simulink model "vibration_harvester"  (R2025b)
settings: Solver=ode23tb  StartTime=0.0  StopTime=10  RelTol=1e-3  AbsTol=1e-6
values from neighbouring files (symbols this model uses):
  alpha = 0.15    [RegenVariables.mat]
  B = 0.05    [RegenVariables.mat]
  C1 = 2000    [RegenVariables.mat]
  C_boost = 0.00047    [RegenVariables.mat]
  C_buck = 0.00022    [RegenVariables.mat]
  cs = 1500    [RegenVariables.mat]
  D = 0.5    [RegenVariables.mat]
  ESR_boost = 3    [RegenVariables.mat]
  ESR_buck = 0.5    [RegenVariables.mat]
  eta = 0.98    [RegenVariables.mat]
  eta_bs = 0.9    [RegenVariables.mat]
  J = 0.01    [RegenVariables.mat]
  Ke = 0.5    [RegenVariables.mat]
  ks = 18000    [RegenVariables.mat]
  Kt = 0.5    [RegenVariables.mat]
  kt = 200000    [RegenVariables.mat]
  L_boost = 0.002    [RegenVariables.mat]
  L_buck = 0.001    [RegenVariables.mat]
  La = 0.005    [RegenVariables.mat]
  ms = 320    [RegenVariables.mat]
  mu = 45    [RegenVariables.mat]
  OCV0 = 3    [RegenVariables.mat]
  OCV_slope = 1.2    [RegenVariables.mat]
  p = 0.005    [RegenVariables.mat]
  Q_nom = 360000    [RegenVariables.mat]
  R0 = 0.05    [RegenVariables.mat]
  R1 = 0.02    [RegenVariables.mat]
  R_load = 50    [RegenVariables.mat]
  Ra = 2    [RegenVariables.mat]
  sigma = 0.002    [RegenVariables.mat]
  SOC0 = 0.5    [RegenVariables.mat]
  v = 20    [RegenVariables.mat]
  v_bat_init = 3.6    [RegenVariables.mat]
libraries: simulink x1
settings Model: NumberOfSteps=1000  Creator=khalid  LastModifiedBy=khalid
settings SolverCC: AutoScaleAbsTol=off

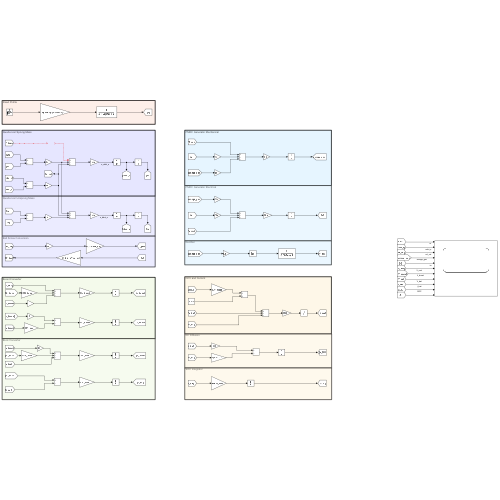
[thumbnail: Simulink's stored preview of the top-level diagram]
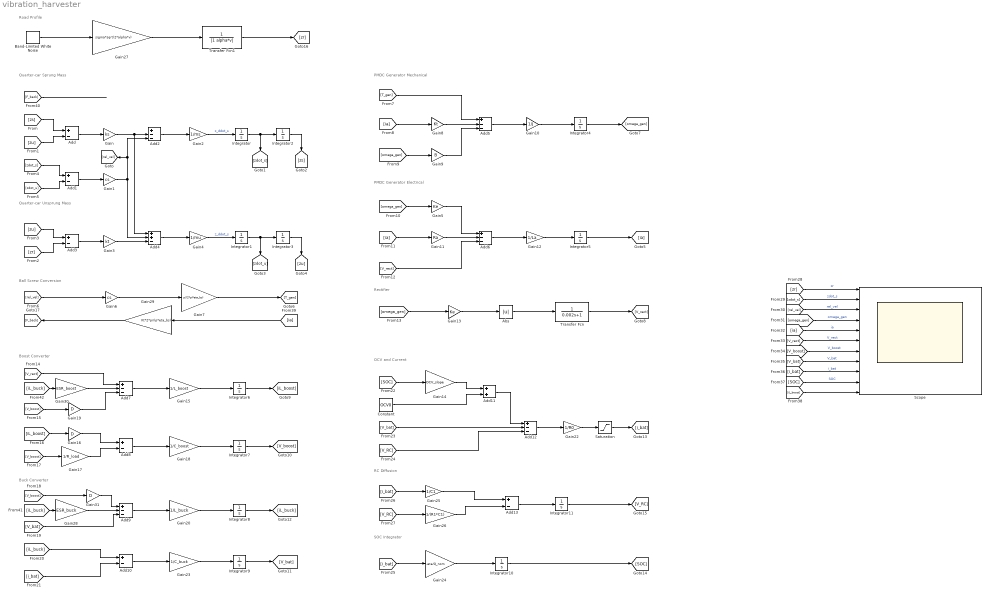
== system vibration_harvester ==
  note: Road Profile
  note: SOC Integrator
  note: RC Diffusion
  note: OCV and Current
  note: Boost Converter
  note: PMDC Generator Mechanical
  note: Ball Screw Conversion
  note: Quarter-car Unsprung Mass
  note: Quarter-car Sprung Mass
  note: PMDC Generator Electrical
  note: Rectifier
  note: Buck Converter
  Abs : Abs  SaturateOnIntegerOverflow=off
  Add{,1,3,8,10,13} (6 alike) : Sum  Inputs=+-
  Add11 : Sum
  Add{2,5..7,9,12} (6 alike) : Sum  Inputs=+--
  Add4 : Sum  Inputs=++-
  Band-Limited White Noise : simulink/Sources/Band-Limited White Noise  Cov=[1]  Ts=0.001  seed=[23341]
  Constant : Constant  Value=OCV0
  Gain : Gain  Gain=ks
  Gain1 : Gain  Gain=cs
  Gain10 : Gain  Gain=1/J
  Gain11 : Gain  Gain=Ra
  Gain12 : Gain  Gain=1/La
  Gain13 : Gain  Gain=Ke
  Gain14 : Gain  Gain=OCV_slope
  Gain15 : Gain  Gain=1/L_boost
  Gain16 : Gain  Gain=D
  Gain17 : Gain  Gain=1/R_load
  Gain18 : Gain  Gain=1/C_boost
  Gain19 : Gain  Gain=D
  Gain2 : Gain  Gain=1/ms
  Gain20 : Gain  Gain=1/L_buck
  Gain22 : Gain  Gain=1/R0
  Gain23 : Gain  Gain=1/C_buck
  Gain24 : Gain  Gain=-eta/Q_nom
  Gain25 : Gain  Gain=1/C1
  Gain26 : Gain  Gain=1/(R1*C1)
  Gain27 : Gain  Gain=sigma*sqrt(2*alpha*v)
  Gain28 : Gain  Gain=ESR_buck
  Gain29 : Gain  Gain=Kt*2*pi/(p*eta_bs)
  Gain3 : Gain  Gain=kt
  Gain30 : Gain  Gain=ESR_boost
  Gain31 : Gain  Gain=D
  Gain4 : Gain  Gain=1/mu
  Gain5 : Gain  Gain=Ke
  Gain6 : Gain  Gain=cs
  Gain7 : Gain  Gain=p/(2*pi*eta_bs)
  Gain8 : Gain  Gain=Kt
  Gain9 : Gain  Gain=B
  Integrator{,1..7,11} (9 alike) : Integrator
  Integrator10 : Integrator  InitialCondition=SOC0  UpperSaturationLimit=1  LowerSaturationLimit=0
  Integrator8 : Integrator  LowerSaturationLimit=0
  Integrator9 : Integrator  InitialCondition=v_bat_init  UpperSaturationLimit=1e9
  Saturation : Saturate  UpperLimit=50  LowerLimit=-10
  Scope : Scope  NumInputPorts=11
      settings: ActiveDisplayString=9  ActiveDisplayYMinimum=-17.5  ActiveDisplayYMaximum=57.5
  Transfer Fcn : TransferFcn  Denominator=[0.002 1]
  Transfer Fcn1 : TransferFcn  Denominator=[1 alpha*v]
  wires:
  [zs] -> Add/1
  [zu] -> Add/2
  Add/1 -> Gain/1
  [zdot_s] -> Add1/1
  [zdot_u] -> Add1/2
  Add1/1 -> Gain1/1
  Gain1/1 -> Add4/2, Add2/3, [rel_vel]
  Gain/1 -> Add4/1, Add2/2
  Add2/1 -> Gain2/1
  Gain2/1 -> Integrator/1  "z_ddot_s"
  Integrator/1 -> Integrator2/1, [zdot_s]
  Integrator2/1 -> [zs]
  Integrator1/1 -> Integrator3/1, [zdot_u]
  Gain4/1 -> Integrator1/1  "z_ddot_s"
  Add4/1 -> Gain4/1
  Gain3/1 -> Add4/3
  Add3/1 -> Gain3/1
  [zu] -> Add3/1
  [zr] -> Add3/2
  [rel_vel] -> Gain6/1
  Gain6/1 -> Gain7/1
  Gain7/1 -> [T_gen]
  [ia] -> Gain8/1
  [omega_gen] -> Gain9/1
  Gain8/1 -> Add5/2
  [T_gen] -> Add5/1
  Gain9/1 -> Add5/3
  Add5/1 -> Gain10/1
  Gain10/1 -> Integrator4/1
  Integrator4/1 -> [omega_gen]
  [omega_gen] -> Gain5/1
  [ia] -> Gain11/1
  Gain11/1 -> Add6/2
  Gain5/1 -> Add6/1
  [V_rect] -> Add6/3
  Add6/1 -> Gain12/1
  Gain12/1 -> Integrator5/1
  Integrator5/1 -> [ia]
  Integrator3/1 -> [zu]
  [omega_gen] -> Gain13/1
  Gain13/1 -> Abs/1
  Abs/1 -> Transfer Fcn/1
  Transfer Fcn/1 -> [V_rect]
  [V_rect] -> Add7/1
  Add7/1 -> Gain15/1
  Gain15/1 -> Integrator6/1
  Integrator6/1 -> [iL_boost]
  [iL_boost] -> Gain16/1
  [V_boost] -> Gain17/1
  Gain16/1 -> Add8/1
  Gain17/1 -> Add8/2
  Add8/1 -> Gain18/1
  Gain18/1 -> Integrator7/1
  Integrator7/1 -> [V_boost]
  Gain20/1 -> Integrator8/1
  Integrator9/1 -> [V_bat]
  [i_bat] -> Add10/2
  Integrator8/1 -> [iL_buck]
  Add10/1 -> Gain23/1
  Gain23/1 -> Integrator9/1
  [iL_buck] -> Add10/1
  Add9/1 -> Gain20/1
  [V_boost] -> Gain31/1
  Gain31/1 -> Add9/1
  [V_boost] -> Gain19/1
  [SOC] -> Gain14/1
  Gain14/1 -> Add11/1
  Constant/1 -> Add11/2
  [V_bat] -> Add12/2
  [V_RC] -> Add12/3
  Add12/1 -> Gain22/1
  [i_bat] -> Gain24/1
  Gain24/1 -> Integrator10/1
  Integrator10/1 -> [SOC]
  [i_bat] -> Gain25/1
  [V_RC] -> Gain26/1
  Gain25/1 -> Add13/1
  Gain26/1 -> Add13/2
  Add13/1 -> Integrator11/1
  Integrator11/1 -> [V_RC]
  Band-Limited White Noise/1 -> Gain27/1
  Gain27/1 -> Transfer Fcn1/1
  Transfer Fcn1/1 -> [zr]
  [zr] -> Scope/1  "zr"
  [zdot_s] -> Scope/2  "zdot_s"
  [rel_vel] -> Scope/3  "rel_vel"
  [omega_gen] -> Scope/4  "omega_gen"
  [ia] -> Scope/5  "ia"
  [V_rect] -> Scope/6  "V_rect"
  [V_boost] -> Scope/7  "V_boost"
  [V_bat] -> Scope/8  "V_bat"
  [i_bat] -> Scope/9  "i_bat"
  [SOC] -> Scope/10  "SOC"
  [iL_boost] -> Scope/11
  Gain29/1 -> [F_back]
  [ia] -> Gain29/1
  Add11/1 -> Add12/1
  [V_bat] -> Add9/3
  Gain28/1 -> Add9/2
  [iL_buck] -> Gain28/1
  [iL_buck] -> Gain30/1
  Gain30/1 -> Add7/2
  Gain19/1 -> Add7/3
  [F_back] -> ?
  ? -> Add2/1
  Saturation/1 -> [i_bat]
  Gain22/1 -> Saturation/1
